simulink model "IVVAN"  (R2022a)
settings: Solver=VariableStepAuto  StartTime=0.0  StopTime=inf  MaxStep=1e-2  RelTol=1e-2
undefined symbols (not defined in the file): CF, Es, Imax, lamda, RaLa, ReLe, Rsh0, Rsh1, Rsh2, step, Stup_osl_polya, Tokivx, Udnom, Vmax, Vnach
libraries: spsSeriesRLCBranchLib x5, spsControlledVoltageSourceLib x3, spsIdealSwitchLib x2, spsCurrentMeasurementLib x2, spsDiodeLib x1, simulink x1, spspowerguiLib x1
settings Model: Creator=Student11  LastModifiedBy=админ
settings SolverCC: AlgebraicLoopSolver=TrustRegion
settings DataIOCC: ReturnWorkspaceOutputs=off
settings DebuggingCC: UnconnectedInputMsg=warning  UnconnectedLineMsg=warning  SFMachineParentedDataDiag=warning  ArithmeticOperatorsInVariantConditions=warning
settings SFSimCC: SimUseLocalCustomCode=off  CustomCodeUndefinedFunction=UseInterfaceOnly
settings RTWCC: RTWUseLocalCustomCode=off
settings CodeAppCC: StateflowObjectComments=on
settings SimscapeCC: SimscapeNormalizeSystem=off

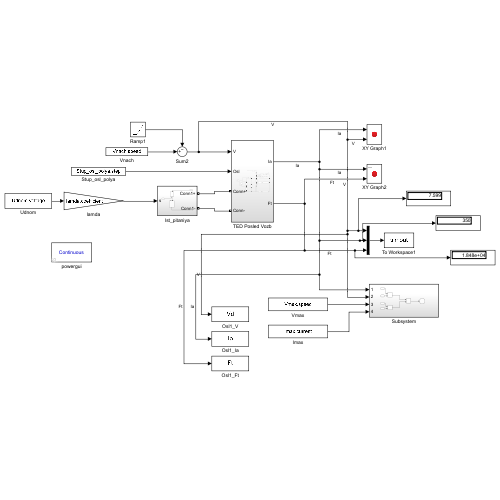
[thumbnail: Simulink's stored preview of the top-level diagram]
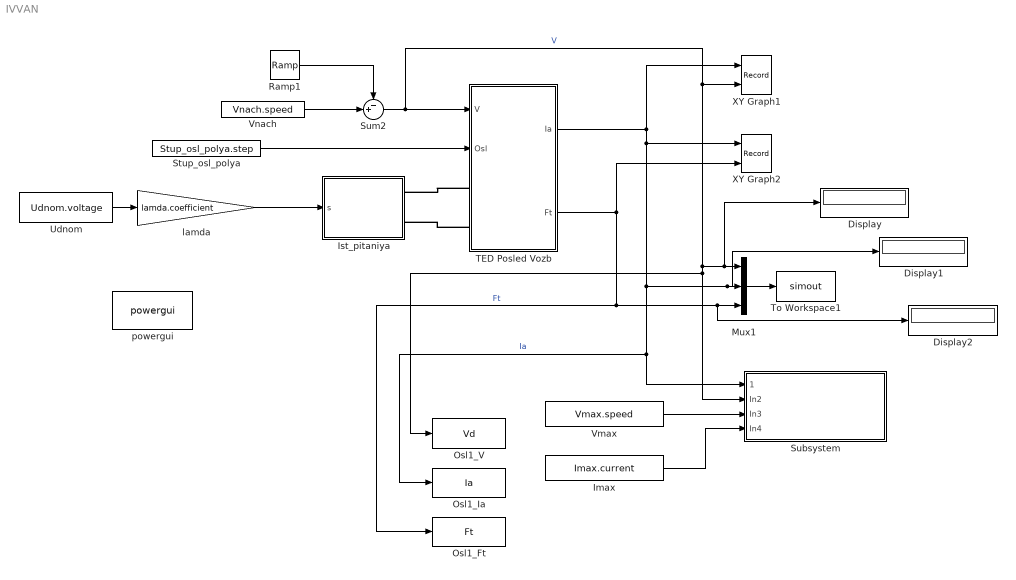
== system IVVAN ==
  Display : Display
  Display1 : Display
  Display2 : Display
  Imax : Constant  Value=Imax.current
  Ist_pitaniya : Subsystem
  Mux1 : Mux  Inputs=3
  Osl1_Ft : ToWorkspace  VariableName=Ft  SampleTime=100
      settings: Save2DSignal=2-D array (concatenate along first dimension)
  Osl1_Ia : ToWorkspace  VariableName=Ia  SampleTime=100
      settings: Save2DSignal=2-D array (concatenate along first dimension)
  Osl1_V : ToWorkspace  VariableName=Vd  SampleTime=10
      settings: Save2DSignal=2-D array (concatenate along first dimension)
  Ramp1 : simulink/Sources/Ramp  slope=0.1  start=0  InitialOutput=0
  Stup_osl_polya : Constant  Value=Stup_osl_polya.step
  Subsystem : Subsystem
  Sum2 : Sum  Inputs=-+|
  TED Posled Vozb : Subsystem
  To Workspace1 : ToWorkspace  VariableName=simout  SaveFormat=Structure  SampleTime=step.measurements
      settings: Save2DSignal=2-D array (concatenate along first dimension)
  Udnom : Constant  Value=Udnom.voltage
  Vmax : Constant  Value=Vmax.speed
  Vnach : Constant  Value=Vnach.speed
  XY Graph1 : Record  FileSettingsInternal="{\"entries\":[{\"content\":{\"excelSettings\":{\"content\":{},\"type\":\"Streamout.ExcelSettings\"}},\"type\":\"Streamout.FileSettingStorage\",\"uuid\":\"b2672be3-39bb-4be8-9488-5323609885ac\"}],\"packageUris\":[\"http://schema.mathworks.com/mf0/streamout_blocks/R2020a\"],\"version\":\"1.0\"}"  Layout=[1 1]  SignalsInternal="{\"entries\":[{\"content\":{\"signals\":[{\"content\":{\"blockPath\":[\"IVVAN/XY Graph1\"],\"channel\":[],\"dimensions\":[1],\"domain\":\"IVVAN/XY Graph1\",\"lineColor\":\"#a2142f\",\"plots\":[1],\"port\":1,\"sid\":[\"\"],\"signalID\":115355,\"signalName\":\"Ia\"},\"type\":\"RecordBlkView.Signal\",\"uuid\":\"154ae224-4333-42da-9b46-673bc796c971\"},{\"content\":{\"blockPath\":[\"IVVAN/XY Graph1\"],\"channel\":[],\"dimensions\":[1],\"domain\":\"IVVAN/XY Graph1\",\"lineColor\":\"#139fff\",\"plots\":[1],\"port\":2,\"sid\":[\"\"],\"signalID\":115359,\"signalName\":\"V\"},\"type\":\"RecordBlkView.Signal\",\"uuid\":\"a272d0e4-812f-492c-9a36-b54a6e59298e\"}]},\"type\":\"RecordBlkView.InputSignals\",\"uuid\":\"83de8d7a-e490-489b-9d4a-07c9416e4977\"}],\"packageUris\":[\"http://schema.mathworks.com/mf0/streamout_blocks/R2020a\"],\"version\":\"1.0\"}"  VisualizationBindings="{\"xyplotplugin\":{\"info\":[{\"series\":[{\"bindingParametersList\":[{\"parameter\":\"X-Axis\",\"signalID\":115359,\"signalName\":\"V\"},{\"parameter\":\"Y-Axis\",\"signalID\":115355,\"signalName\":\"Ia\"}],\"seriesID\":11720}],\"subplotID\":1}]}}"  CompatibilityTag=XY  st=-1
  XY Graph2 : Record  FileSettingsInternal="{\"entries\":[{\"content\":{\"excelSettings\":{\"content\":{},\"type\":\"Streamout.ExcelSettings\"}},\"type\":\"Streamout.FileSettingStorage\",\"uuid\":\"c3af5991-73d9-42a9-bf75-c09cdf38dab6\"}],\"packageUris\":[\"http://schema.mathworks.com/mf0/streamout_blocks/R2020a\"],\"version\":\"1.0\"}"  Layout=[1 1]  SignalsInternal="{\"entries\":[{\"content\":{\"signals\":[{\"content\":{\"blockPath\":[\"IVVAN/XY Graph2\"],\"channel\":[],\"dimensions\":[1],\"domain\":\"IVVAN/XY Graph2\",\"lineColor\":\"#22b573\",\"plots\":[1],\"port\":1,\"sid\":[\"\"],\"signalID\":115363,\"signalName\":\"Ia\"},\"type\":\"RecordBlkView.Signal\",\"uuid\":\"d0d4de56-479f-4dc7-891a-78d36490e771\"},{\"content\":{\"blockPath\":[\"IVVAN/XY Graph2\"],\"channel\":[],\"dimensions\":[1],\"domain\":\"IVVAN/XY Graph2\",\"lineColor\":\"#0072bd\",\"plots\":[1],\"port\":2,\"sid\":[\"\"],\"signalID\":115367,\"signalName\":\"Ft\"},\"type\":\"RecordBlkView.Signal\",\"uuid\":\"fb9d33f6-971b-4e2f-beb0-3b2dde9289a6\"}]},\"type\":\"RecordBlkView.InputSignals\",\"uuid\":\"a2de2db7-16e0-449a-970f-ac06e1038a8a\"}],\"packageUris\":[\"http://schema.mathworks.com/mf0/streamout_blocks/R2020a\"],\"version\":\"1.0\"}"  VisualizationBindings="{\"xyplotplugin\":{\"info\":[{\"series\":[{\"bindingParametersList\":[{\"parameter\":\"X-Axis\",\"signalID\":115367,\"signalName\":\"Ft\"},{\"parameter\":\"Y-Axis\",\"signalID\":115363,\"signalName\":\"Ia\"}],\"seriesID\":42676}],\"subplotID\":1}]}}"  CompatibilityTag=XY  st=-1
  lamda : Gain  Gain=lamda.coefficient
  powergui : spspowerguiLib/powergui  Priority=1  SimulationMode=Continuous  SampleTime=50e-6  frequency=60  Iterations=50  frequencyindice=0  Pbase=100e6  ErrMax=1e-4  UnitsV=kV  UnitsW=MW  buscounter=0  FunctionMessages=off  echomessages=off  EnableUseOfTLC=off  CurrentSourceSwitches=off  DisableSnubberDevices=off  DisableRonSwitches=off  DisableVfSwitches=off  DisplayEquations=off  AutomaticDiscreteSolvers=off  SolverType=Tustin/Backward Euler (TBE)  Interpol=off  ExternalGateDelay=off  methode=off  Ts=100  x0status=blocks  SPID=on  SwTol=0  HookPort=off  NonlinearTolerance=1e-4  nMaxIteration=100  ContinueOnMaxIteration=off  RestoreLinks=warning  ResistiveCurrentMeasurement=off  Frange=[0:2:500]  Ylog=off  Xlog=on  ShowGrid=off  save=off  variable=ZData  structure=0  ZoomFFT=off  StartTime=0.0  cycles=1  DisplayStyle=1  fundamental=60  FreqAxis=off  MaxFrequency=1000  frequencyindicesteady=1  RmsSteady=1  display=off
  wires:
  Udnom/1 -> lamda/1
  lamda/1 -> Ist_pitaniya/1(s)
  Stup_osl_polya/1 -> TED Posled Vozb/2(Osl)
  Sum2/1 -> XY Graph1/2, Display/1, Mux1/1, Osl1_V/1, Subsystem/2(In2), TED Posled Vozb/1(V)  "V"
  Ramp1/1 -> Sum2/1
  Vnach/1 -> Sum2/2
  Mux1/1 -> To Workspace1/1
  TED Posled Vozb/1(Ia) -> XY Graph1/1, Display1/1, Mux1/2, Osl1_Ia/1, Subsystem/1(1), XY Graph2/1  "Ia"
  TED Posled Vozb/2(Ft) -> XY Graph2/2, Osl1_Ft/1, Display2/1, Mux1/3  "Ft"
  Imax/1 -> Subsystem/4(In4)
  Vmax/1 -> Subsystem/3(In3)
  connections:
  TED Posled Vozb/LConn1 -- Ist_pitaniya/RConn1
  TED Posled Vozb/LConn2 -- Ist_pitaniya/RConn2

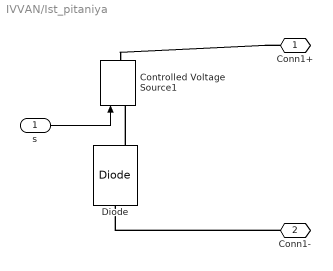
== system IVVAN/Ist_pitaniya ==
  s : Inport
  Controlled Voltage Source1 : spsControlledVoltageSourceLib/Controlled Voltage Source  Initialize=on  Source_Type=AC  Amplitude=0  Phase=0  Frequency=0  Measurements=None
  Diode : spsDiodeLib/Diode  Ron=0.001  Lon=0  Vf=0.8  IC=0  UseSnubber=0  Rs=500  Cs=250e-9  Measurements=on
  Conn1+ : PMIOPort  Side=Right
  Conn1- : PMIOPort  Port=2  Side=Right
  wires:
  s/1 -> Controlled Voltage Source1/1
  connections:
  Conn1-/RConn1 -- Diode/LConn1
  Diode/RConn1 -- Controlled Voltage Source1/LConn1
  Conn1+/RConn1 -- Controlled Voltage Source1/RConn1

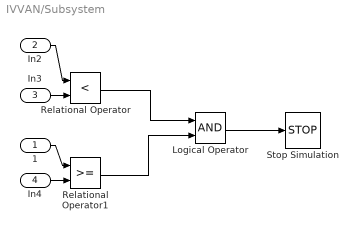
== system IVVAN/Subsystem ==
  1 : Inport
  In2 : Inport  Port=2
  In3 : Inport  Port=3
  In4 : Inport  Port=4
  Logical Operator : Logic  AllPortsSameDT=off  OutDataTypeStr=boolean
  Relational Operator : RelationalOperator  Operator=<  OutDataTypeStr=boolean  RndMeth=Simplest  InputSameDT=off
  Relational Operator1 : RelationalOperator  OutDataTypeStr=boolean  RndMeth=Simplest  InputSameDT=off
  Stop Simulation : Stop
  wires:
  Relational Operator/1 -> Logical Operator/1
  Relational Operator1/1 -> Logical Operator/2
  In2/1 -> Relational Operator/1
  Logical Operator/1 -> Stop Simulation/1
  1/1 -> Relational Operator1/1
  In4/1 -> Relational Operator1/2
  In3/1 -> Relational Operator/2

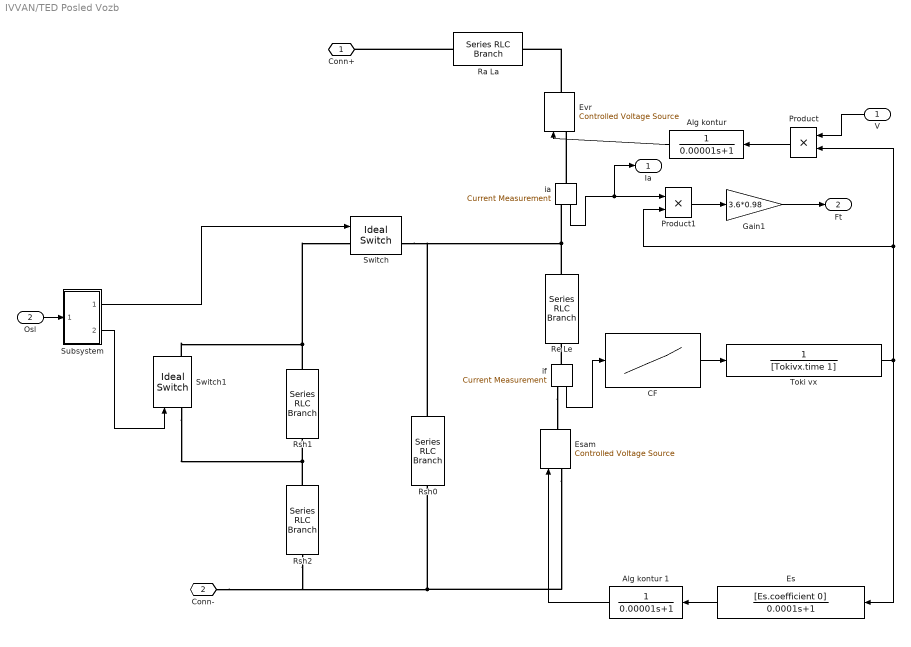
== system IVVAN/TED Posled Vozb ==
  V : Inport
  Osl : Inport  Port=2
  Alg kontur : TransferFcn  Denominator=[0.00001 1]
  Alg kontur 1 : TransferFcn  Denominator=[0.00001 1]
  CF : Lookup_n-D  NumberOfTableDimensions=1  BreakpointsForDimension1=CF.currentvozb  Table=CF.CvF  InternalRulePriority=Speed  RndMeth=Simplest
  Es : TransferFcn  Numerator=[Es.coefficient 0]  Denominator=[0.0001 1]
  Esam : spsControlledVoltageSourceLib/Controlled Voltage Source  Initialize=on  Source_Type=AC  Amplitude=0  Phase=0  Frequency=0  Measurements=None
  Evr : spsControlledVoltageSourceLib/Controlled Voltage Source  Initialize=on  Source_Type=AC  Amplitude=0  Phase=0  Frequency=0  Measurements=None
  Gain1 : Gain  Gain=3.6*0.98
  Product : Product
  Product1 : Product
  Ra La : spsSeriesRLCBranchLib/Series RLC Branch  LConnTagsString=__new0  RConnTagsString=__new0  BranchType=RL  Resistance=RaLa.Res  Inductance=RaLa.Ind  SetiL0=off  InitialCurrent=0  Capacitance=1e-6  Setx0=off  InitialVoltage=0  Measurements=None
  Re Le : spsSeriesRLCBranchLib/Series RLC Branch  LConnTagsString=__new0  RConnTagsString=__new0  BranchType=RL  Resistance=ReLe.Res  Inductance=ReLe.Ind  SetiL0=off  InitialCurrent=0  Capacitance=1e-6  Setx0=off  InitialVoltage=0  Measurements=None
  Rsh0 : spsSeriesRLCBranchLib/Series RLC Branch  LConnTagsString=__new0  RConnTagsString=__new0  BranchType=R  Resistance=Rsh0.Res  Inductance=1e-3  SetiL0=off  InitialCurrent=0  Capacitance=1e-6  Setx0=off  InitialVoltage=0  Measurements=None
  Rsh1 : spsSeriesRLCBranchLib/Series RLC Branch  LConnTagsString=__new0  RConnTagsString=__new0  BranchType=R  Resistance=Rsh1.Res  Inductance=1e-3  SetiL0=off  InitialCurrent=0  Capacitance=1e-6  Setx0=off  InitialVoltage=0  Measurements=None
  Rsh2 : spsSeriesRLCBranchLib/Series RLC Branch  LConnTagsString=__new0  RConnTagsString=__new0  BranchType=R  Resistance=Rsh2.Res  Inductance=1e-3  SetiL0=off  InitialCurrent=0  Capacitance=1e-6  Setx0=off  InitialVoltage=0  Measurements=None
  Subsystem : Subsystem
  Switch : spsIdealSwitchLib/Ideal Switch  Ron=0.001  Lon=0  IC=0  Rs=1e5  Cs=inf  Measurements=on
  Switch1 : spsIdealSwitchLib/Ideal Switch  Ron=0.001  Lon=0  IC=0  Rs=1e5  Cs=inf  Measurements=on
  Toki vx : TransferFcn  Denominator=[Tokivx.time 1]
  ia : spsCurrentMeasurementLib/Current Measurement  PhasorSimulation=off  OutputType=Complex  PSBequivalent=0
  if : spsCurrentMeasurementLib/Current Measurement  PhasorSimulation=off  OutputType=Complex  PSBequivalent=0
  Conn+ : PMIOPort  Side=Left
  Conn- : PMIOPort  Port=2  Side=Left
  Ia : Outport
  Ft : Outport  Port=2
  wires:
  Osl/1 -> Subsystem/1(In1)
  Alg kontur/1 -> Evr/1
  Product/1 -> Alg kontur/1
  Alg kontur 1/1 -> Esam/1
  Product1/1 -> Gain1/1
  Gain1/1 -> Ft/1
  Toki vx/1 -> Es/1, Product1/2, Product/2
  CF/1 -> Toki vx/1
  if/1 -> CF/1
  ia/1 -> Ia/1, Product1/1
  Es/1 -> Alg kontur 1/1
  V/1 -> Product/1
  Subsystem/1(Out1) -> Switch/1
  Subsystem/2(Out2) -> Switch1/1
  connections:
  Rsh1/LConn1 -- Switch1/RConn1 -- Switch/LConn1
  Esam/LConn1 -- Rsh0/RConn1 -- Rsh2/RConn1 -- Conn-/RConn1
  ia/LConn1 -- Evr/LConn1
  Rsh2/LConn1 -- Switch1/LConn1 -- Rsh1/RConn1
  if/RConn1 -- Esam/RConn1
  if/LConn1 -- Re Le/RConn1
  Ra La/LConn1 -- Conn+/RConn1
  Evr/RConn1 -- Ra La/RConn1
  Re Le/LConn1 -- Rsh0/LConn1 -- Switch/RConn1 -- ia/RConn1

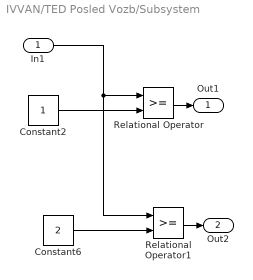
== system IVVAN/TED Posled Vozb/Subsystem ==
  In1 : Inport
  Constant2 : Constant
  Constant6 : Constant  Value=2
  Relational Operator : RelationalOperator  OutDataTypeStr=boolean  RndMeth=Simplest  InputSameDT=off
  Relational Operator1 : RelationalOperator  OutDataTypeStr=boolean  RndMeth=Simplest  InputSameDT=off
  Out1 : Outport
  Out2 : Outport  Port=2
  wires:
  Constant6/1 -> Relational Operator1/2
  In1/1 -> Relational Operator/1, Relational Operator1/1
  Relational Operator/1 -> Out1/1
  Constant2/1 -> Relational Operator/2
  Relational Operator1/1 -> Out2/1
